simulink model "NavFilterTestHarness21"  (Simulink 7.9)
settings: Solver=FixedStepDiscrete  StartTime=min(IMUtime)  StopTime=max(IMUtime)  FixedStep=0.001  RelTol=1e-3
undefined symbols (not defined in the file or in its folder): accel, ADSframe, ADStime, angRate, ATTframe, CourseDeg, GndSpd, GPSframe, GPStime, Hgt, IMUframe, IMUtime, LatDeg, LngDeg, MagBiasX, MagBiasY, MagBiasZ, MAGframe, MAGtime, MagX, MagY, MagZ, Pitch, Roll, Veas, VelD, Yaw
libraries: simulink x13
(part 2 of 5)

== system NavFilterTestHarness21/WatchDog/Get AHRS Data/wrapAng to +-pi ==
  In1 : Inport  OutDataTypeStr=single
  If : If  IfExpression=u1 > single(pi)
  If Action Subsystem : Subsystem  TreatAsAtomicUnit=on
  If Action Subsystem1 : Subsystem  TreatAsAtomicUnit=on
  Merge : Merge
  Out1 : Outport  OutDataTypeStr=single
  wires:
  In1/1 -> If Action Subsystem1/1(In1), If Action Subsystem/1(In1), If/1
  If/2 -> If Action Subsystem/Action
  If/1 -> If Action Subsystem1/Action
  If Action Subsystem/1(Out1) -> Merge/1
  If Action Subsystem1/1(Out1) -> Merge/2
  Merge/1 -> Out1/1

== system NavFilterTestHarness21/InertialNavFilter/CalculateInitialStates/Read AHRS solution/wrapAng to +-pi ==
  In1 : Inport  OutDataTypeStr=single
  If : If  IfExpression=u1 > single(pi)
  If Action Subsystem : Subsystem  TreatAsAtomicUnit=on
  If Action Subsystem1 : Subsystem  TreatAsAtomicUnit=on
  Merge : Merge
  Out1 : Outport  OutDataTypeStr=single
  wires:
  In1/1 -> If Action Subsystem1/1(In1), If Action Subsystem/1(In1), If/1
  If/2 -> If Action Subsystem/Action
  If/1 -> If Action Subsystem1/Action
  If Action Subsystem/1(Out1) -> Merge/1
  If Action Subsystem1/1(Out1) -> Merge/2
  Merge/1 -> Out1/1

== system NavFilterTestHarness21/LogData/GetReferenceData/wrapAng to +-pi/If Action Subsystem ==
  In1 : Inport
  Action Port : ActionPort  ActionType=else
  Out1 : Outport
  wires:
  In1/1 -> Out1/1

== system NavFilterTestHarness21/LogData/GetReferenceData/wrapAng to +-pi/If Action Subsystem1 ==
  In1 : Inport
  Action Port : ActionPort  ActionType=then
  Add : Sum  Inputs=+-
  Constant : Constant  Value=2*pi  OutDataTypeStr=single
  Out1 : Outport
  wires:
  In1/1 -> Add/1
  Add/1 -> Out1/1
  Constant/1 -> Add/2

== system NavFilterTestHarness21/WatchDog/Get AHRS Data/wrapAng to +-pi/If Action Subsystem ==
  In1 : Inport
  Action Port : ActionPort  ActionType=else
  Out1 : Outport
  wires:
  In1/1 -> Out1/1

== system NavFilterTestHarness21/WatchDog/Get AHRS Data/wrapAng to +-pi/If Action Subsystem1 ==
  In1 : Inport
  Action Port : ActionPort  ActionType=then
  Add : Sum  Inputs=+-
  Constant : Constant  Value=2*pi  OutDataTypeStr=single
  Out1 : Outport
  wires:
  In1/1 -> Add/1
  Add/1 -> Out1/1
  Constant/1 -> Add/2

== system NavFilterTestHarness21/InertialNavFilter/CalculateInitialStates/Read AHRS solution/wrapAng to +-pi/If Action Subsystem ==
  In1 : Inport
  Action Port : ActionPort  ActionType=else
  Out1 : Outport
  wires:
  In1/1 -> Out1/1

== system NavFilterTestHarness21/InertialNavFilter/CalculateInitialStates/Read AHRS solution/wrapAng to +-pi/If Action Subsystem1 ==
  In1 : Inport
  Action Port : ActionPort  ActionType=then
  Add : Sum  Inputs=+-
  Constant : Constant  Value=2*pi  OutDataTypeStr=single
  Out1 : Outport
  wires:
  In1/1 -> Add/1
  Add/1 -> Out1/1
  Constant/1 -> Add/2

== matlab function WatchDog/wrapAnglePi ==
  data: angleOut output double; angleIn input double
function angleOut   = wrapAnglePi(angleIn)
%#codegen

if abs(angleIn) <= pi
    angleOut = angleIn;
elseif  angleIn < -pi
    angleOut = angleIn + 2*pi;
elseif angleIn > pi
    angleOut = angleIn - 2*pi;
else
    angleOut = angleIn;
end

end

== matlab function InertialNavFilter/Predict States ==
  data: nextStates output double; correctedDelAng output double; correctedDelVel output double; accNavMag output double; states input double; gravityNED input double; earthRateNED input double; angRate input double; accel input double; dt input double
%#codegen
function [nextStates,correctedDelAng,correctedDelVel,accNavMag]  = UpdateStrapdownEquationsNED( ...
    states, ...
    gravityNED, ...
    earthRateNED, ...
    angRate, ...
    accel, ...
    dt)

% Define parameters used for previous angular rates and acceleration shwich
% are used for trapezoidal integration
persistent prevAngRate;
if isempty(prevAngRate)
    prevAngRate = angRate;
end
persistent prevAccel;
if isempty(prevAccel)
    prevAccel = accel;
end
% define persistent variables for previous delta angle and velocity which
% are required for sculling and coning error corrections
persistent prevDelAng;
if isempty(prevDelAng)
    prevDelAng = single([0;0;0]);
end
persistent prevDelVel;
if isempty(prevDelVel)
    prevDelVel = single([0;0;0]);
end
persistent Tbn;
if isempty(Tbn)
    Tbn = single(eye(3));
end

% Convert IMU data to delta angles and velocities using trapezoidal
% integration
dAng = 0.5*(angRate + prevAngRate)*dt;
dVel = 0.5*(accel   + prevAccel  )*dt;
prevAngRate = angRate;
prevAccel   = accel;

% Remove sensor bias errors
dAng = dAng - states(11:13);

% Apply rotational and skulling corrections
correctedDelVel= dVel + ...
    0.5*cross(prevDelAng + dAng , prevDelVel + dVel) + 1/6*cross(prevDelAng + dAng , cross(prevDelAng + dAng , prevDelVel + dVel)) + ... % rotational correction
    1/12*(cross(prevDelAng , dVel) + cross(prevDelVel , dAng)); % sculling correction

% Apply corrections for earths rotation rate and coning errors
correctedDelAng   = dAng - transpose(Tbn)*earthRateNED*dt + 1/12*cross(prevDelAng , dAng);

% Save current measurements
prevDelAng = dAng;
prevDelVel = dVel;

% Initialise the updated state vector
nextStates   = states;

% Convert the rotation vector to its equivalent quaternion
rotationMag = sqrt(correctedDelAng(1)^2 + correctedDelAng(2)^2 + correctedDelAng(3)^2);
if rotationMag<1e-12
  deltaQuat = single([1;0;0;0]);
else
  deltaQuat = [cos(0.5*rotationMag); correctedDelAng/rotationMag*sin(0.5*rotationMag)];
end

% Update the quaternions by rotating from the previous attitude through
% the delta angle rotation quaternion
qUpdated = [states(1)*deltaQuat(1)-transpose(states(2:4))*deltaQuat(2:4); states(1)*deltaQuat(2:4) + deltaQuat(1)*states(2:4) + cross(states(2:4),deltaQuat(2:4))];

% Normalise the quaternions and update the quaternion states
quatMag = sqrt(qUpdated(1)^2 + qUpdated(2)^2 + qUpdated(3)^2 + qUpdated(4)^2);
if (quatMag < 1e-16)
    nextStates(1:4) = qUpdated;
else
    nextStates(1:4) = qUpdated / quatMag;
end

% Calculate the body to nav cosine matrix
Tbn = [nextStates(1)^2 + nextStates(2)^2 - nextStates(3)^2 - nextStates(4)^2, 2*(nextStates(2)*nextStates(3) - nextStates(1)*nextStates(4)), 2*(nextStates(2)*nextStates(4) + nextStates(1)*nextStates(3));...
      2*(nextStates(2)*nextStates(3) + nextStates(1)*nextStates(4)), nextStates(1)^2 - nextStates(2)^2 + nextStates(3)^2 - nextStates(4)^2, 2*(nextStates(3)*nextStates(4) - nextStates(1)*nextStates(2));...
      2*(nextStates(2)*nextStates(4)-nextStates(1)*nextStates(3)), 2*(nextStates(3)*nextStates(4) + nextStates(1)*nextStates(2)), nextStates(1)^2 - nextStates(2)^2 - nextStates(3)^2 + nextStates(4)^2];
  
% transform body delta velocities to delta velocities in the nav frame
delVelNav = Tbn * correctedDelVel + gravityNED*dt;

% calculate the magnitude of the nav acceleration (required for GPS
% variance estimation)
accNavMag = sqrt(delVelNav(1)^2 + delVelNav(2)^2 + delVelNav(3)^2) / dt;

% If calculating position save previous velocity
lastVelocity = nextStates(5:7);

% Sum delta velocities to get velocity after removing gravitational skew and correcting for transport rate
nextStates(5:7) = states(5:7) + delVelNav;


% If calculating postions, do a trapezoidal integration for position
nextStates(8:10)     = states(8:10) + 0.5*(nextStates(5:7) + lastVelocity)*dt;

% Copy the remaining states across
nextStates(11:21) = states(11:21);

end
